simulink model "p8"  (R2020a)
settings: Solver=VariableStepAuto  StartTime=0.0  StopTime=10  RelTol=1e-3
settings Model: Creator=007  LastModifiedBy=007

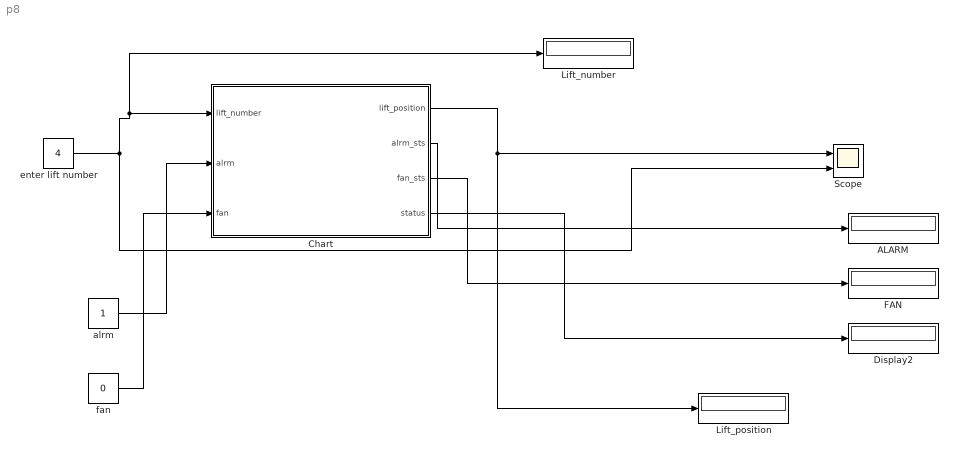
== system p8 ==
  ALARM : Display
  Chart : Stateflow chart  TreatAsAtomicUnit=on
  Display2 : Display
  FAN : Display
  Lift_number : Display
  Lift_position : Display
  Scope : Scope  NumInputPorts=2
  alrm : Constant
  enter lift number : Constant  Value=4
  fan : Constant  Value=0
  wires:
  enter lift number/1 -> Lift_number/1, Chart/1(lift_number), Scope/2
  Chart/1(lift_position) -> Lift_position/1, Scope/1
  alrm/1 -> Chart/2(alrm)
  fan/1 -> Chart/3(fan)
  Chart/2(alrm_sts) -> ALARM/1
  Chart/3(fan_sts) -> FAN/1
  Chart/4(status) -> Display2/1

== stateflow chart p8/Chart ==
  state LIFT
    entry:
    status=1;
    state second_floor
      entry:
      lift_position=2;
    state third_floor
      entry:
      lift_position=3;
    state first_floor
      entry:
      lift_position=1;
    state ON
      entry:
      lift_position=0;
    state fourth_floor
      entry:
      lift_position=4;
    state fifth_floor1
      entry:
      lift_position=5;
    ON -> first_floor [order 3] : [lift_number==1]
    ON -> second_floor [order 1] : [lift_number==2]
    ON -> third_floor [order 2] : [lift_number==3]
    (default) -> ON
    ON -> fifth_floor1 [order 4] : [lift_number==5]
    ON -> fourth_floor [order 5] : [lift_number==4]
  state ALARM
    entry:
    alrm_sts=0;
    state alarm_on
      entry:
      alrm_sts=1;
    (default) -> alarm_on
  state FAN
    entry:
    fan_sts=0;
    state Fan_on
      entry:
      fan_sts=1;
    (default) -> Fan_on
  (default) -> LIFT [order 1]
  (default) -> ALARM [order 2]
  LIFT -> alarm_on [order 1] : [alrm==1]
  (default) -> FAN [order 3]
  LIFT -> FAN [order 2] : [fan==1]
  data: lift_position output; lift_number input; alrm input; fan input; alrm_sts output; fan_sts output; status output
